simulink model "DC_Motor_System_2025b"  (R2025b)
settings: Solver=ode23t  StartTime=0.0  StopTime=10  FixedStep=Ts  RelTol=1e-7  EnableMultiTasking=on
libraries: simulink_extras x2
settings Model: Creator=SABA  LastModifiedBy=Murl0
settings SolverCC: ZeroCrossAlgorithm=Adaptive  AlgebraicLoopSolver=TrustRegion
settings DataIOCC: LimitDataPoints=on  SaveFormat=Array  ReturnWorkspaceOutputs=off
settings OptimizationCC: LifeSpan=inf
settings DebuggingCC: IgnoredZcDiagnostic=none  UnconnectedInputMsg=warning  UnconnectedOutputMsg=warning  UnconnectedLineMsg=warning  SFUnexpectedBacktrackingDiag=warning  SFNoUnconditionalDefaultTransitionDiag=warning  SFExecutionAtInitializationDiag=none  ArithmeticOperatorsInVariantConditions=warning
settings HardwareCC: ProdBitPerPointer=32.0  ProdBitPerSizeT=32.0  ProdBitPerPtrDiffT=32.0  ProdLargestAtomicFloat=None  ProdIntDivRoundTo=Undefined  ProdEndianess=Unspecified  ProdWordSize=32.0  ProdHWDeviceType=32-bit Generic
settings ModelReferenceCC: PropagateSignalLabelsOutOfModel=off
settings SFSimCC: SimUseLocalCustomCode=off  CustomCodeUndefinedFunction=UseInterfaceOnly
settings RTWCC: RTWUseLocalCustomCode=off  GPUComputeCapability=3.5
settings CodeAppCC: StateflowObjectComments=on
settings GRTTargetCC: TargetLangStandard=C89/C90 (ANSI)
settings ConfigComp: CovMetricSettings=dw  CovSaveCumulativeToWorkspaceVar=on  CovSaveSingleToWorkspaceVar=on  CovExternalEMLEnable=off

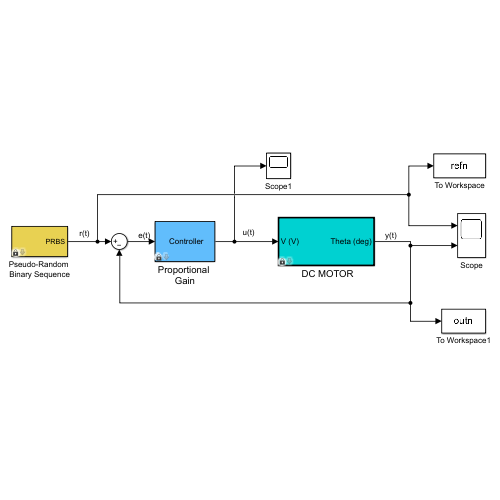
[thumbnail: Simulink's stored preview of the top-level diagram]
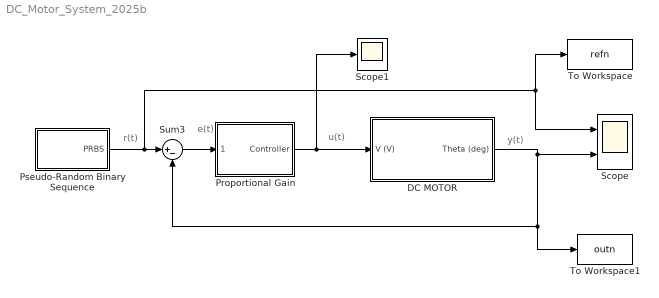
== system DC_Motor_System_2025b ==
  note: u(t)
  note: y(t)
  note: r(t)
  note: e(t)
  " DC MOTOR" : Subsystem  TreatAsAtomicUnit=on  mask(DC Servo Motor Module){La=0.15*10^-3, Ra=3, Jm=2.47*10^-7, Bm=1.2319*10^-7, noise=1}
      mask prompts: La "Armature Inductance - La (H)"; Ra "Armature Resistance - Ra (ohm)"; Jm "Motor Inertia - Jm (oz.in.sec^2)"; Bm "Motor Viscous Friction - Bm (N.m.sec)"; noise "Additive Noise (ON = 1, OFF = 0)"
      mask help: The DC Motor model with dead-zone nonlinearities.
      settings: MinAlgLoopOccurrences=on
  Proportional Gain : Subsystem  mask(Controller){Kp=1}
      mask prompts: Kp "Proportional Gain (Kp)"
      mask help: Proportional Controller with saturated output. The output limited between -1.4V to +1.4V
      mask DialogControl Parameters Prompt: Parameters
  Pseudo-Random Binary Sequence : Subsystem  mask(DPRBS){N=2000, K=80, A=35}
      mask prompts: N "Number of Sample Points (N)"; K "Switch Constant (K)"; A "Amplitude (A)"
      mask help: Generates a random switching sequence of discrete samples valued at -A and +A.
  Scope : Scope  NumInputPorts=2
      settings: TimeSpan=20  Title=Reference Signal  ActiveDisplayYMinimum=-43.75  ActiveDisplayYMaximum=43.75  YLabel=Amplitude (deg)  DataLoggingSaveFormat=Array
  Scope1 : Scope
      settings: Title=Control Signal (V)  ActiveDisplayYMinimum=-1.5712603761640918  ActiveDisplayYMaximum=1.5572958175479286
  Sum3 : Sum  Inputs=|+-
  To Workspace : ToWorkspace  VariableName=refn  SampleTime=1/150
  To Workspace1 : ToWorkspace  VariableName=outn  SampleTime=1/150
  wires:
  Sum3/1 -> Proportional Gain/1("  ")
  Pseudo-Random Binary Sequence/1(PRBS) -> Scope/1, To Workspace/1, Sum3/1
  " DC MOTOR"/1(Theta (deg)) -> Scope/2, To Workspace1/1, Sum3/2
  Proportional Gain/1("Controller    ") -> Scope1/1, " DC MOTOR"/1(V (V))

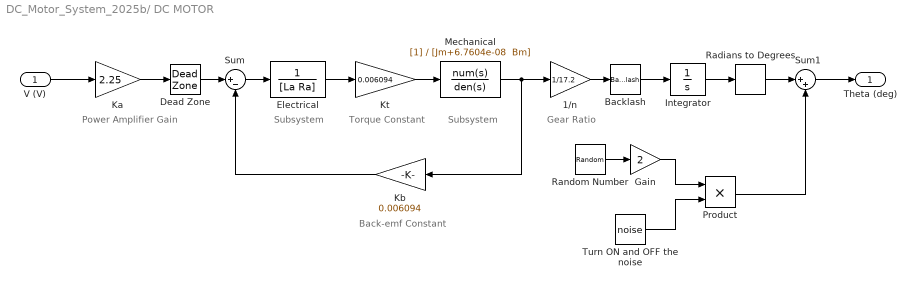
== system DC_Motor_System_2025b/ DC MOTOR ==
  note: Gear Ratio
  note: Subsystem
  note: Subsystem
  note: Power Amplifier
      |          Gain
  note: Back-emf Constant
  note: Torque Constant
  V (V) : Inport
  1/n : Gain  Gain=1/17.2
  Backlash : Backlash  BacklashWidth=0.03  ZeroCross=off
  Dead Zone : DeadZone  LowerValue=-0.05  UpperValue=0.05  ZeroCross=off
  Electrical : TransferFcn  Denominator=[La Ra]
  Gain : Gain  Gain=2
  Integrator : TransferFcn  Denominator=[1 0]
  Ka : Gain  Gain=2.25
  Kb : Gain  Gain=0.006094
  Kt : Gain  Gain=0.006094
  Mechanical : TransferFcn  Denominator="[Jm+6.7604e-08  Bm]"
  Product : Product
  Radians to Degrees : simulink_extras/Transformations/Radians to Degrees
  Random Number : RandomNumber  Seed=randi([0 100],1,1)  SampleTime=1/150
  Sum : Sum  Inputs=|+-
  Sum1 : Sum  Inputs=|++
  Turn ON and OFF the noise : Constant  Value=noise  SampleTime=1/150
  Theta (deg) : Outport
  wires:
  Sum/1 -> Electrical/1
  Integrator/1 -> Radians to Degrees/1
  Electrical/1 -> Kt/1
  Kt/1 -> Mechanical/1
  Mechanical/1 -> Kb/1, 1/n/1
  1/n/1 -> Backlash/1
  Kb/1 -> Sum/2
  Ka/1 -> Dead Zone/1
  V (V)/1 -> Ka/1
  Dead Zone/1 -> Sum/1
  Radians to Degrees/1 -> Sum1/1
  Sum1/1 -> Theta (deg)/1
  Random Number/1 -> Gain/1
  Turn ON and OFF the noise/1 -> Product/2
  Product/1 -> Sum1/2
  Backlash/1 -> Integrator/1
  Gain/1 -> Product/1

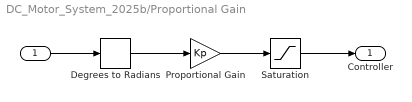
== system DC_Motor_System_2025b/Proportional Gain ==
  "  " : Inport
  Degrees to Radians : simulink_extras/Transformations/Degrees to Radians
  Proportional Gain : Gain  Gain=Kp
  Saturation : Saturate  UpperLimit=1.4  LowerLimit=-1.4  ZeroCross=off
  "Controller    " : Outport
  wires:
  "  "/1 -> Degrees to Radians/1
  Proportional Gain/1 -> Saturation/1
  Degrees to Radians/1 -> Proportional Gain/1
  Saturation/1 -> "Controller    "/1

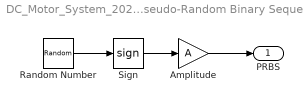
== system DC_Motor_System_2025b/Pseudo-Random Binary Sequence ==
  Amplitude : Gain  Gain=A
  Random Number : RandomNumber  Seed=randi([0 100],1,1)  SampleTime=10*K/N
  Sign : Signum
  PRBS : Outport
  wires:
  Sign/1 -> Amplitude/1
  Random Number/1 -> Sign/1
  Amplitude/1 -> PRBS/1
